simulink model "persistent_test"  (R2022b)
settings: Solver=FixedStepDiscrete  StartTime=0.0  StopTime=10.0  RelTol=1e-3  EnableMultiTasking=on
PostLoadFcn:
  | disp('---- model PostLoadFcn ----');
  | mbd_diag_init(struct('snapSignal',mbd_diag_init().snapSignal+1))
InitFcn:
  | disp('---- model InitFcn ----');
  | mbd_diag_init(struct('snapSignal',mbd_diag_init().snapSignal+1))
libraries: MbdLib_Required x1
settings Model: Creator=KenYoshioka  LastModifiedBy=KenYoshioka
settings SolverCC: AutoInsertRateTranBlk=on
settings OptimizationCC: DefaultParameterBehavior=Inlined  DefaultUnderspecifiedDataType=single  EnhancedBackFolding=on  BooleansAsBitfields=on  PassReuseOutputArgsAs=Individual arguments  ZeroExternalMemoryAtStartup=off  ZeroInternalMemoryAtStartup=off  OptimizeBlockOrder=speed  DifferentSizesBufferReuse=on  EfficientTunableParamExpr=on
settings DebuggingCC: ParameterTunabilityLossMsg=error
settings HardwareCC: ProdBitPerPointer=32  ProdBitPerSizeT=32  ProdBitPerPtrDiffT=32  ProdLargestAtomicInteger=Long  ProdLargestAtomicFloat=Double  ProdWordSize=32  ProdHWDeviceType=ARM Compatible->ARM Cortex
settings ModelReferenceCC: ModelReferenceNumInstancesAllowed=Single
settings SFSimCC: MATLABDynamicMemAlloc=off
settings RTWCC: Description=MBD Embedded Target SAME70 Cortex M7 (real-time)  SystemTargetFile=MBD_SAME70_stf.tlc  TemplateMakefile=MBD_SAME70.tmf  Toolchain=xc32 - v3.01
settings CodeAppCC: ForceParamTrailComments=on  IgnoreCustomStorageClasses=off  MaxIdLength=255  OperatorAnnotations=on  SimulinkDataObjDesc=on  SFDataObjDesc=on  InsertBlockDesc=on
settings STFCustomTargetCC: MultiwordLength=256  IncludeMdlTerminateFcn=off  CombineOutputUpdateFcns=on  CombineSignalStateStructs=on  SuppressErrorStatus=on  ERTCustomFileBanners=on  SupportContinuousTime=off  RemoveResetFunc=on  MATLABClassNameForMDSCustomization=Simulink.SoftwareTarget.ERTCustomization  UseToolchainInfoCompliant=on  SystemTargetFile=MBD_SAME70_stf.tlc
settings ERTTargetCC: ParMdlRefBuildCompliant=off  CompOptLevelCompliant=off  ConcurrentExecutionCompliant=off  IncludeMdlTerminateFcn=off  CombineSignalStateStructs=on  SuppressErrorStatus=on  SupportNonInlinedSFcns=on  ModelStepFunctionPrototypeControlCompliant=off  CPPClassGenCompliant=off  ExtModeStaticAllocSize=2000  InlinedParameterPlacement=NonHierarchical  ERTCustomFileTemplate=mbd_lib_interface.tlc  MaxLineWidth=110

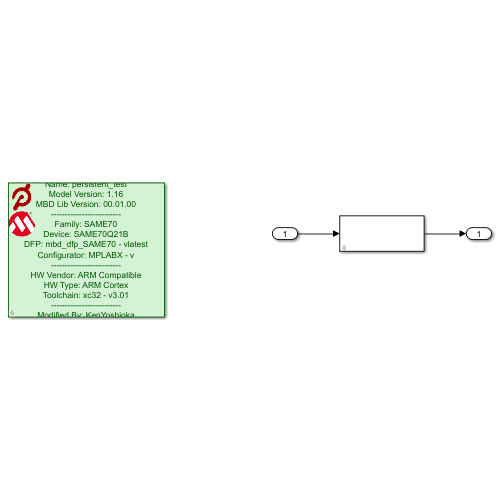
[thumbnail: Simulink's stored preview of the top-level diagram]
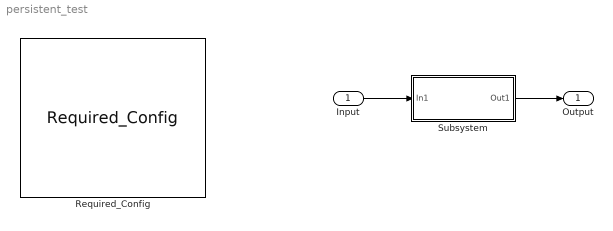
== system persistent_test ==
  Input : Inport
  Required_Config : MbdLib_Required/Required_Config  Tag=MBD_Target_Info  Param_update=1
      settings: SourceProductName=Peloton Interface Library
  Subsystem : Subsystem  LoadFcn=|  InitFcn=|
      LoadFcn=|
      | disp('---- block LoadFcn ----');
      | mbd_diag_init(struct('snapSignal',mbd_diag_init().snapSignal+1))
      InitFcn=|
      | disp('---- block InitFcn ----');
      | mbd_diag_init(struct('snapSignal',mbd_diag_init().snapSignal+1))
      mask init:
      | disp('---- initialization ----');
      | mbd_diag_init(struct('portalParam',mbd_diag_init().portalParam+1))
      mask Display:
      | disp_in_icon('---- icon ----');
      | mbd_diag_init(struct('portalSignal',mbd_diag_init().portalSignal+1))
  Output : Outport
  wires:
  Input/1 -> Subsystem/1(In1)
  Subsystem/1(Out1) -> Output/1

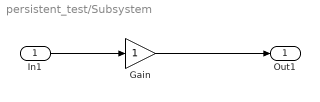
== system persistent_test/Subsystem ==
  In1 : Inport
  Gain : Gain
  Out1 : Outport
  wires:
  In1/1 -> Gain/1
  Gain/1 -> Out1/1
